simulink model "hydraulic_act_systems"  (R2013a)
settings: Solver=ode23t  StartTime=0.0  StopTime=10.0  FixedStep=1e-4  RelTol=1e-3
model workspace (MATLAB code in the model file):
  | % Data obtained from:
  | % ------------------------------------------------------------
  | % HyQ-Robot: Standard Definition for Joint Angles
  | % and Kinematic Parameters of the Legs and Torso
  | %
  | % Project: HyQ-Robot V1.0 with Leg V2.0
  | % Genoa, 9th July 2010
  | %-------------------------------------------------------------
  | % This Matlab file was made by:
  | % Job Ledezma
  | % Genova, Feb 2016
  | %-------------------------------------------------------------
  | 
  | 
  | % ________________________________________
  | %
  | %                HYL DESCRIPTION PARAMETERS
  | %________________________________________
  | 
  | % ---- Leg data ------
  | 
  | m1 = 1.772;              % Kg - Upper leg mass
  | m2 = 0.808;              % Kg - Lower leg mass
  | M = 3.982;                % Kg - Base mass
  | P_01 = 0.08;             % m - distance P0-P1
  | P_12 = 0.350;           % m - distance P1-P2
  | P_23 = 0.330;           % m - distance P2-P3
  | FR = 0.02;                 % m - foot radius
  | P1m1 = 0.164;           % m - distance P1-Pm1
  | P2m2 = 0.122;           % m - distance P2-Pm2
  | I1zz = 0.0713;           % kg·m2 - Inertia upper leg
  | I2zz = 0.0218;           % kg·m2 - Inertia lower leg
  | em1 = deg2rad(7.9);  % rad
  | em2 = deg2rad(0);     % rad
  | g  = 9.810;                 % m/s2 - gravity
  | 
  | % ----- Lever Arm Parameters -----
  | 
  | % Hip joint
  | a1   = 0.3219;             % m
  | b1   = 0.045;               % m
  | e11 = deg2rad(6.24); % rad
  | e12 = deg2rad(0);      % rad
  | 
  | % Knee joint
  | a2 = 0.3218;               % m
  | b2 = 0.045;                 % m
  | e21 = deg2rad(8.04);  % rad
  | e22 = deg2rad(6);       % rad
  | 
  | % ----- Limit Angles --------
  | 
  | % Initial conditions
  | q0_0 = 1;                           % m - height of the floating base
  | q1_0 = deg2rad(45);         % rad - HFE angle
  | q2_0 = deg2rad(-90);        % rad - KFE angle
  | 
  | % Max angle limits
  | q1Max = deg2rad(70);       % rad
  | q2Max = deg2rad(-20);      % rad
  | 
  | % Min angle limits
  | q1Min = deg2rad(-50);        % rad
  | q2Min = deg2rad(-140);      % rad
  | q0Min = P_01+P_12*cos(q1Min)+P_23*cos(q1Min+q2Min)+FR;     % m
  | 
  | % ________________________________________________________
  | %
  | %                                        HYDRAULIC PARAMETERS
  | % ________________________________________________________
  | 
  | % ------ Power unit --------
  | 
  | ps  = 160e5;                            % Pa - Supply pressure
  | pt  = 10e5;                              % Pa - Tank pressure
  | dpt = ps - pt;                           % Pa - Delta pressure
  | beta = 1.4e9;                          % Pa- Effective bulk modulus
  | 
  | % Initial condition for integrators
  | xo = 0;
  | 
  | pAo = 0;%ps/2;
  | pBo = 0;%ps/2;
  | 
  | %----- Cylinder - HOERBIGER LB6 16 10 0080 4M ----------
  | 
  | Dp = 0.016;                             % m - Piston diameter
  | Dr = 0.010;                              % m - Rod diameter
  | L  = 0.080;                               % m- Stroke
  | Aa = pi*(Dp^2)/4;                   % m^2 - Area A of the piston
  | Ab = pi*(Dp^2-Dr^2)/4;         % m^2 - Area B of the piston
  | r  = Aa/Ab;                              % Relation between areas
  | fv = 700;                                 %  Ns/m - Viscous friction
  | leak =1.7*10^-13;                 % m3/(s.Pa) - Cylinder leakage
  | Mp = ((pi*Dr^2/4)*L + Aa*0.15)*7860;    % Kg - Piston mass (approximated)
  | Lcyl = 0.280;                           % m - Total length of the cylinder
  | 
  | %-----  Valve Parameters - MOOG E024 - 177LA ----------
  | 
  | In   = 10;                               % I - Nominal control current
  | Qn   = 7.5 / 60e3;                 % m^3/s - Nominal flow rate
  | dptn = 70e5;                         % Pa - Valve pressure drop
  | Qlk   = 0.375 / 60e3;               % m^3/s - Leakage flow
  | Plk    = 70e5;                       % Pa - Nominal supply pressure for leakage test
  | wn    = 2*100*pi;                    % rad/s - Valve's natural frequency
  | E       = 0.7;                           % Valve's damping coefficient
  | Kv     = Qn/sqrt(dptn);          % m^3/(s*sqrt(Pa)) - Total flow coefficient
  | Kva    = Kv*sqrt(2);               % m^3/(s*sqrt(Pa)) - Partial flow coefficient A
  | Kvb    = Kv*sqrt(2);               % m^3/(s*sqrt(Pa)) - Partial flow coefficient B
  | Kvlk   = Qlk/sqrt(2*Plk);         % m^3/(s*sqrt(Pa)) - Total leakage flow coefficient
  | KvlkA  = Kvlk;                         % m^3/(s*sqrt(Pa)) -  Partial leakage flow coefficient A
  | KvlkB  = Kvlk;                         % m^3/(s*sqrt(Pa)) - Partial leakage flow coefficient B
  | up_dz = 0;                             % V - Upper limit of dead zone
  | lw_dz = 0;                              % V - Lower limit of dead zone
  | 
  | %------------   Manifold  -----------
  | % Review this part with the manifold's CAD design
  | 
  | v1a = (pi*(0.0035^2)/4)*0.07255;
  | v2a = (pi*(0.006^2)/4)*(0.090-0.012);
  | v1b = (pi*(0.0035^2)/4)*0.04491;
  | v2b = (pi*(0.006^2)/4)*(0.019+0.009);
  | v3b = (pi*(0.006^2)/4)*(0.007+0.009);
  | V0A = v1a + v2a;                                            % Dead volume coupled to chamber A
  | V0B = v1b + v2b + v3b;                                  % Dead volume coupled to chamber B
  | 
  | %-------  Load cell - BURSTER 8417-6005 ----------
  | 
  | xs = 20e-6;                            % m - Maximum deflection @ full scale
  | Fs = 5000;                             % N - Maximum force
  | Ks = Fs / xs ;                         % N·m - Load cell stiffness
  | 
  | noise = 0;                            %N - noise due nonlinearities, hysteresis, non repeatibility
  | 
  | %------ Accumulator - FOX-ITALY HST 0,04 ----------
  | 
  | acc = 0;
  | 
  | n = 1.4;                                % Polytropic constant
  | V0 = 0.04e-3;                       % m3 - Initial volume
  | P0 = 100e5 + 1e5;               % Pa - Precharge pressure
libraries: sdolib x4
settings Model: Creator=Toshiba  LastModifiedBy=Toshiba
settings SolverCC: ZeroCrossAlgorithm=Adaptive

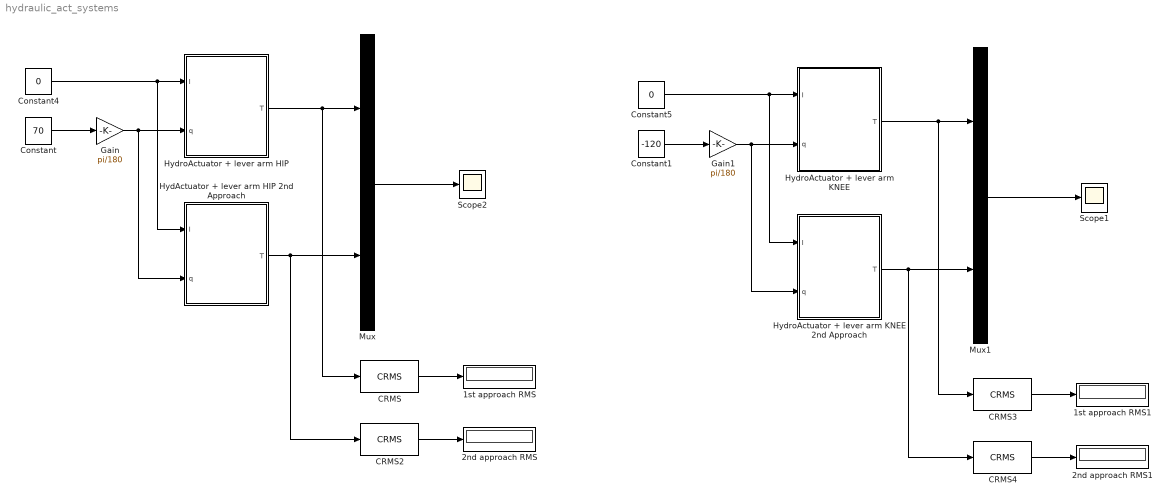
== system hydraulic_act_systems ==
  1st approach RMS : Display
  1st approach RMS1 : Display
  2nd approach RMS : Display
  2nd approach RMS1 : Display
  CRMS{,2..4} (4 alike) : sdolib/RMS Blocks/CRMS
  Constant : Constant  Value=70
  Constant1 : Constant  Value=-120
  Constant4 : Constant  Value=0
  Constant5 : Constant  Value=0
  Gain : Gain  Gain=pi/180
  Gain1 : Gain  Gain=pi/180
  HydActuator + lever arm HIP 2nd Approach : Subsystem
  HydroActuator + lever arm HIP : Subsystem
  HydroActuator + lever arm KNEE : Subsystem
  HydroActuator + lever arm KNEE 2nd Approach : Subsystem
  Mux : Mux  Inputs=2
  Mux1 : Mux  Inputs=2
  Scope1 : Scope
      settings: YMin=-152500  YMax=-117500
  Scope2 : Scope
      settings: YMin=-152500  YMax=-117500  SaveName=ScopeData2
  wires:
  Constant/1 -> Gain/1
  Gain/1 -> HydActuator + lever arm HIP 2nd Approach/2(q), HydroActuator + lever arm HIP/2(q)
  Constant1/1 -> Gain1/1
  Gain1/1 -> HydroActuator + lever arm KNEE 2nd Approach/2(q), HydroActuator + lever arm KNEE/2(q)
  Constant4/1 -> HydActuator + lever arm HIP 2nd Approach/1(I), HydroActuator + lever arm HIP/1(I)
  Constant5/1 -> HydroActuator + lever arm KNEE 2nd Approach/1(I), HydroActuator + lever arm KNEE/1(I)
  HydroActuator + lever arm HIP/1(T) -> CRMS/1, Mux/1
  HydActuator + lever arm HIP 2nd Approach/1(T) -> CRMS2/1, Mux/2
  Mux/1 -> Scope2/1
  HydroActuator + lever arm KNEE/1(T) -> CRMS3/1, Mux1/1
  HydroActuator + lever arm KNEE 2nd Approach/1(T) -> CRMS4/1, Mux1/2
  CRMS/1 -> 1st approach RMS/1
  Mux1/1 -> Scope1/1
  CRMS2/1 -> 2nd approach RMS/1
  CRMS3/1 -> 1st approach RMS1/1
  CRMS4/1 -> 2nd approach RMS1/1

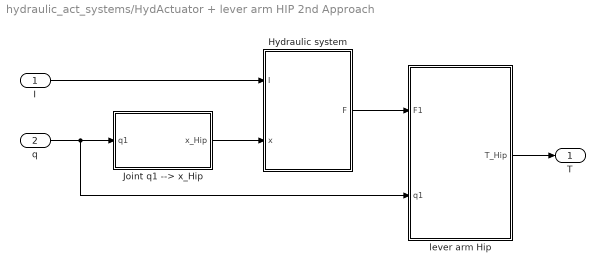
== system hydraulic_act_systems/HydActuator + lever arm HIP 2nd Approach ==
  I : Inport
  q : Inport  Port=2
  Hydraulic system : Subsystem
  "Joint q1 --> x_Hip  " : MATLAB Function  TreatAsAtomicUnit=on
  lever arm Hip : MATLAB Function  TreatAsAtomicUnit=on
  T : Outport
  wires:
  q/1 -> "Joint q1 --> x_Hip  "/1(q1), lever arm Hip/2(q1)
  I/1 -> Hydraulic system/1(I)
  lever arm Hip/1(T_Hip) -> T/1
  Hydraulic system/1(F) -> lever arm Hip/1(F1)
  "Joint q1 --> x_Hip  "/1(x_Hip) -> Hydraulic system/2(x)

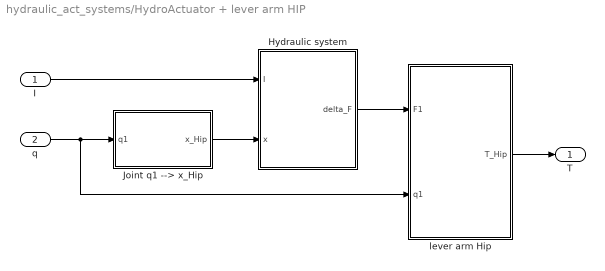
== system hydraulic_act_systems/HydroActuator + lever arm HIP ==
  I : Inport
  q : Inport  Port=2
  Hydraulic system : Subsystem
  "Joint q1 --> x_Hip  " : MATLAB Function  TreatAsAtomicUnit=on
  lever arm Hip : MATLAB Function  TreatAsAtomicUnit=on
  T : Outport
  wires:
  "Joint q1 --> x_Hip  "/1(x_Hip) -> Hydraulic system/2(x)
  Hydraulic system/1(delta_F) -> lever arm Hip/1(F1)
  lever arm Hip/1(T_Hip) -> T/1
  I/1 -> Hydraulic system/1(I)
  q/1 -> lever arm Hip/2(q1), "Joint q1 --> x_Hip  "/1(q1)

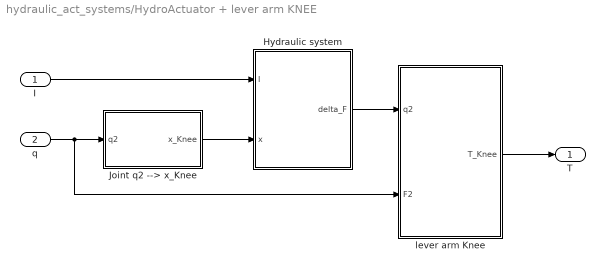
== system hydraulic_act_systems/HydroActuator + lever arm KNEE ==
  I : Inport
  q : Inport  Port=2
  Hydraulic system : Subsystem
  Joint q2 --> x_Knee : MATLAB Function  TreatAsAtomicUnit=on
  lever arm Knee : MATLAB Function  TreatAsAtomicUnit=on
  T : Outport
  wires:
  q/1 -> lever arm Knee/2(F2), Joint q2 --> x_Knee/1(q2)
  Joint q2 --> x_Knee/1(x_Knee) -> Hydraulic system/2(x)
  Hydraulic system/1(delta_F) -> lever arm Knee/1(q2)
  I/1 -> Hydraulic system/1(I)
  lever arm Knee/1(T_Knee) -> T/1

== system hydraulic_act_systems/HydroActuator + lever arm KNEE 2nd Approach ==
  I : Inport
  q : Inport  Port=2
  Hydraulic system : Subsystem
  Joint q2 --> x_Knee : MATLAB Function  TreatAsAtomicUnit=on
  lever arm Knee : MATLAB Function  TreatAsAtomicUnit=on
  T : Outport
  wires:
  lever arm Knee/1(T_Knee) -> T/1
  I/1 -> Hydraulic system/1(I)
  Hydraulic system/1(F) -> lever arm Knee/1(q2)
  Joint q2 --> x_Knee/1(x_Knee) -> Hydraulic system/2(x)
  q/1 -> Joint q2 --> x_Knee/1(q2), lever arm Knee/2(F2)

== system hydraulic_act_systems/HydActuator + lever arm HIP 2nd Approach/Hydraulic system ==
  I : Inport
  x : Inport  Port=2
  Cylinder HOERBIGER LB6 1610 0080 4M : Subsystem
  Servovalve MOOG E024-177LA : Subsystem
  F : Outport
  wires:
  Servovalve MOOG E024-177LA/2(qB) -> Cylinder HOERBIGER LB6 1610 0080 4M/2(qB)
  Servovalve MOOG E024-177LA/1(qA) -> Cylinder HOERBIGER LB6 1610 0080 4M/1(qA)
  Cylinder HOERBIGER LB6 1610 0080 4M/2(pA) -> Servovalve MOOG E024-177LA/2(pA)
  Cylinder HOERBIGER LB6 1610 0080 4M/3(pB) -> Servovalve MOOG E024-177LA/3(pB)
  I/1 -> Servovalve MOOG E024-177LA/1(I)
  Cylinder HOERBIGER LB6 1610 0080 4M/1(F) -> F/1
  x/1 -> Cylinder HOERBIGER LB6 1610 0080 4M/3(x)

== system hydraulic_act_systems/HydroActuator + lever arm HIP/Hydraulic system ==
  I : Inport
  x : Inport  Port=2
  Cylinder HOERBIGER LB6 1610 0080 4M : Subsystem
  Servovalve MOOG E024-177LA : Subsystem
  delta_F : Outport
  wires:
  Servovalve MOOG E024-177LA/2(qB) -> Cylinder HOERBIGER LB6 1610 0080 4M/2(qB)
  Servovalve MOOG E024-177LA/1(qA) -> Cylinder HOERBIGER LB6 1610 0080 4M/1(qA)
  Cylinder HOERBIGER LB6 1610 0080 4M/2(pA1) -> Servovalve MOOG E024-177LA/2(pA)
  Cylinder HOERBIGER LB6 1610 0080 4M/3(pB1) -> Servovalve MOOG E024-177LA/3(pB)
  I/1 -> Servovalve MOOG E024-177LA/1(I)
  Cylinder HOERBIGER LB6 1610 0080 4M/1(delta_F) -> delta_F/1
  x/1 -> Cylinder HOERBIGER LB6 1610 0080 4M/3(x)

== system hydraulic_act_systems/HydroActuator + lever arm KNEE/Hydraulic system ==
  I : Inport
  x : Inport  Port=2
  Cylinder HOERBIGER LB6 1610 0080 4M : Subsystem
  Servovalve MOOG E024-177LA : Subsystem
  delta_F : Outport
  wires:
  Servovalve MOOG E024-177LA/2(qB) -> Cylinder HOERBIGER LB6 1610 0080 4M/2(qB)
  Servovalve MOOG E024-177LA/1(qA) -> Cylinder HOERBIGER LB6 1610 0080 4M/1(qA)
  Cylinder HOERBIGER LB6 1610 0080 4M/2(pA1) -> Servovalve MOOG E024-177LA/2(pA)
  Cylinder HOERBIGER LB6 1610 0080 4M/3(pB1) -> Servovalve MOOG E024-177LA/3(pB)
  I/1 -> Servovalve MOOG E024-177LA/1(I)
  Cylinder HOERBIGER LB6 1610 0080 4M/1(delta_F) -> delta_F/1
  x/1 -> Cylinder HOERBIGER LB6 1610 0080 4M/3(x)

== system hydraulic_act_systems/HydroActuator + lever arm KNEE 2nd Approach/Hydraulic system ==
  I : Inport
  x : Inport  Port=2
  Cylinder HOERBIGER LB6 1610 0080 4M : Subsystem
  Servovalve MOOG E024-177LA : Subsystem
  F : Outport
  wires:
  Servovalve MOOG E024-177LA/2(qB) -> Cylinder HOERBIGER LB6 1610 0080 4M/2(qB)
  Servovalve MOOG E024-177LA/1(qA) -> Cylinder HOERBIGER LB6 1610 0080 4M/1(qA)
  Cylinder HOERBIGER LB6 1610 0080 4M/2(pA) -> Servovalve MOOG E024-177LA/2(pA)
  Cylinder HOERBIGER LB6 1610 0080 4M/3(pB) -> Servovalve MOOG E024-177LA/3(pB)
  I/1 -> Servovalve MOOG E024-177LA/1(I)
  Cylinder HOERBIGER LB6 1610 0080 4M/1(F) -> F/1
  x/1 -> Cylinder HOERBIGER LB6 1610 0080 4M/3(x)

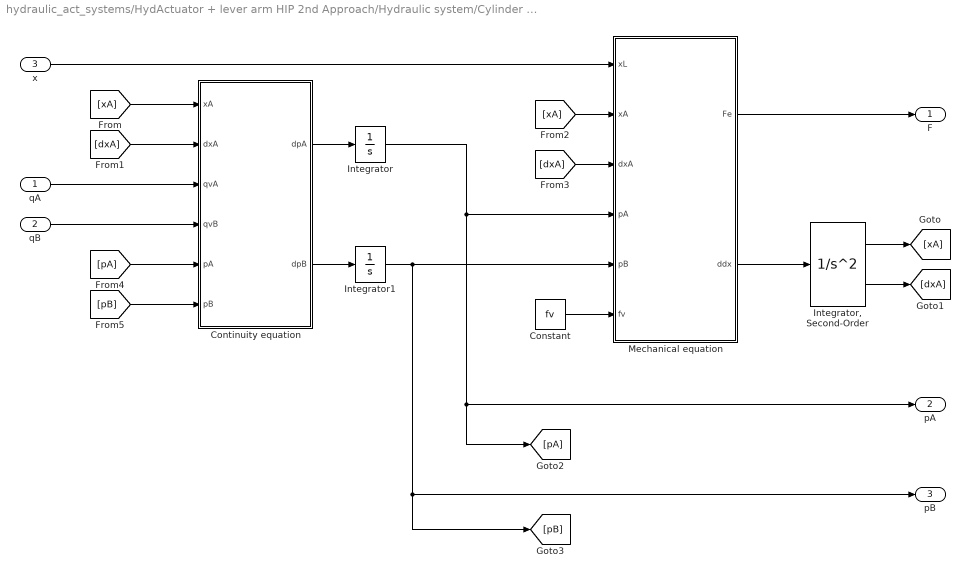
== system hydraulic_act_systems/HydActuator + lever arm HIP 2nd Approach/Hydraulic system/Cylinder HOERBIGER LB6 1610 0080 4M ==
  qA : Inport
  qB : Inport  Port=2
  x : Inport  Port=3
  Constant : Constant  Value=fv
  Continuity equation : MATLAB Function  TreatAsAtomicUnit=on
  Integrator : Integrator  InitialCondition=pAo
  "Integrator, Second-Order" : SecondOrderIntegrator  ICX=xo  LimitX=on  UpperLimitX=L  LowerLimitX=0
  Integrator1 : Integrator  InitialCondition=pBo
  Mechanical equation : MATLAB Function  TreatAsAtomicUnit=on
  F : Outport
  pA : Outport  Port=2
  pB : Outport  Port=3
  wires:
  Continuity equation/1(dpA) -> Integrator/1
  Continuity equation/2(dpB) -> Integrator1/1
  Integrator/1 -> [pA], pA/1, Mechanical equation/4(pA)
  Integrator1/1 -> pB/1, [pB], Mechanical equation/5(pB)
  qA/1 -> Continuity equation/3(qvA)
  qB/1 -> Continuity equation/4(qvB)
  Mechanical equation/2(ddx) -> "Integrator, Second-Order"/1
  [dxA] -> Continuity equation/2(dxA)
  [xA] -> Continuity equation/1(xA)
  "Integrator, Second-Order"/1 -> [xA]
  "Integrator, Second-Order"/2 -> [dxA]
  Constant/1 -> Mechanical equation/6(fv)
  [xA] -> Mechanical equation/2(xA)
  [dxA] -> Mechanical equation/3(dxA)
  [pA] -> Continuity equation/5(pA)
  [pB] -> Continuity equation/6(pB)
  Mechanical equation/1(Fe) -> F/1
  x/1 -> Mechanical equation/1(xL)

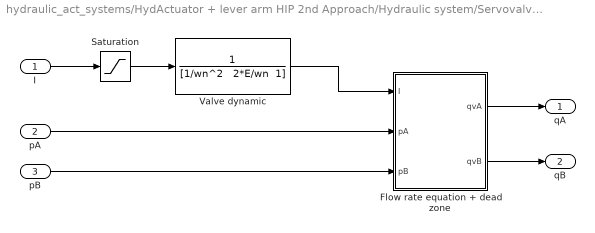
== system hydraulic_act_systems/HydActuator + lever arm HIP 2nd Approach/Hydraulic system/Servovalve MOOG E024-177LA ==
  I : Inport
  pA : Inport  Port=2
  pB : Inport  Port=3
  Flow rate equation + dead zone : MATLAB Function  TreatAsAtomicUnit=on
  Saturation : Saturate  UpperLimit=In  LowerLimit=-In  LinearizeAsGain=off
  Valve dynamic : TransferFcn  Numerator=1  Denominator="[1/wn^2   2*E/wn  1]"
  qA : Outport
  qB : Outport  Port=2
  wires:
  Saturation/1 -> Valve dynamic/1
  I/1 -> Saturation/1
  Valve dynamic/1 -> Flow rate equation + dead zone/1(I)
  pA/1 -> Flow rate equation + dead zone/2(pA)
  pB/1 -> Flow rate equation + dead zone/3(pB)
  Flow rate equation + dead zone/2(qvB) -> qB/1
  Flow rate equation + dead zone/1(qvA) -> qA/1

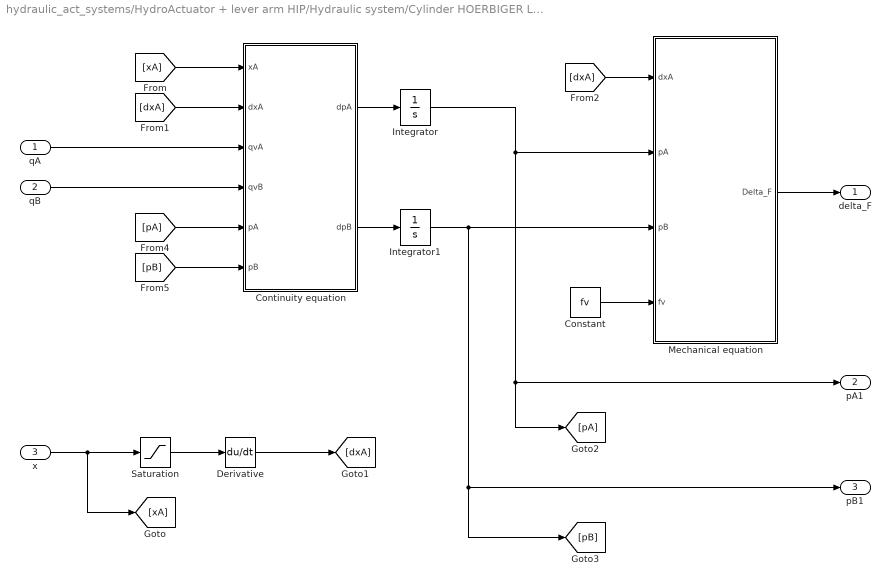
== system hydraulic_act_systems/HydroActuator + lever arm HIP/Hydraulic system/Cylinder HOERBIGER LB6 1610 0080 4M ==
  qA : Inport
  qB : Inport  Port=2
  x : Inport  Port=3
  Constant : Constant  Value=fv
  Continuity equation : MATLAB Function  TreatAsAtomicUnit=on
  Derivative : Derivative
  Integrator : Integrator  InitialCondition=pAo
  Integrator1 : Integrator  InitialCondition=pBo
  Mechanical equation : MATLAB Function  TreatAsAtomicUnit=on
  Saturation : Saturate  UpperLimit=L  LowerLimit=0
  delta_F : Outport
  pA1 : Outport  Port=2
  pB1 : Outport  Port=3
  wires:
  Continuity equation/1(dpA) -> Integrator/1
  Continuity equation/2(dpB) -> Integrator1/1
  qA/1 -> Continuity equation/3(qvA)
  qB/1 -> Continuity equation/4(qvB)
  [dxA] -> Continuity equation/2(dxA)
  [xA] -> Continuity equation/1(xA)
  Constant/1 -> Mechanical equation/4(fv)
  Derivative/1 -> [dxA]
  Mechanical equation/1(Delta_F) -> delta_F/1
  x/1 -> [xA], Saturation/1
  Saturation/1 -> Derivative/1
  [dxA] -> Mechanical equation/1(dxA)
  Integrator/1 -> [pA], pA1/1, Mechanical equation/2(pA)
  Integrator1/1 -> [pB], pB1/1, Mechanical equation/3(pB)
  [pA] -> Continuity equation/5(pA)
  [pB] -> Continuity equation/6(pB)

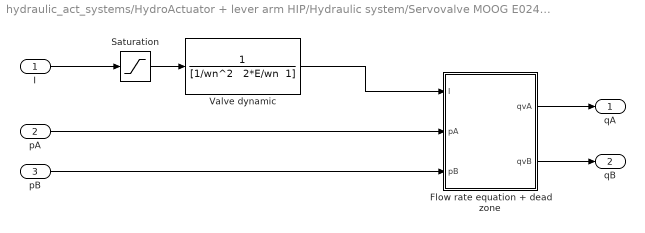
== system hydraulic_act_systems/HydroActuator + lever arm HIP/Hydraulic system/Servovalve MOOG E024-177LA ==
  I : Inport
  pA : Inport  Port=2
  pB : Inport  Port=3
  Flow rate equation + dead zone : MATLAB Function  TreatAsAtomicUnit=on
  Saturation : Saturate  UpperLimit=In  LowerLimit=-In  LinearizeAsGain=off
  Valve dynamic : TransferFcn  Numerator=1  Denominator="[1/wn^2   2*E/wn  1]"
  qA : Outport
  qB : Outport  Port=2
  wires:
  Saturation/1 -> Valve dynamic/1
  I/1 -> Saturation/1
  Valve dynamic/1 -> Flow rate equation + dead zone/1(I)
  pA/1 -> Flow rate equation + dead zone/2(pA)
  pB/1 -> Flow rate equation + dead zone/3(pB)
  Flow rate equation + dead zone/2(qvB) -> qB/1
  Flow rate equation + dead zone/1(qvA) -> qA/1

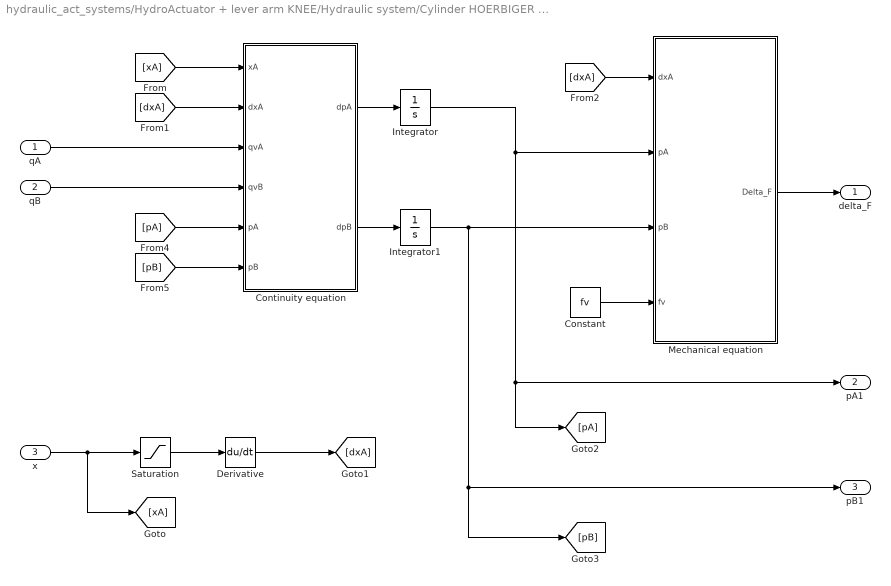
== system hydraulic_act_systems/HydroActuator + lever arm KNEE/Hydraulic system/Cylinder HOERBIGER LB6 1610 0080 4M ==
  qA : Inport
  qB : Inport  Port=2
  x : Inport  Port=3
  Constant : Constant  Value=fv
  Continuity equation : MATLAB Function  TreatAsAtomicUnit=on
  Derivative : Derivative
  Integrator : Integrator  InitialCondition=pAo
  Integrator1 : Integrator  InitialCondition=pBo
  Mechanical equation : MATLAB Function  TreatAsAtomicUnit=on
  Saturation : Saturate  UpperLimit=L  LowerLimit=0
  delta_F : Outport
  pA1 : Outport  Port=2
  pB1 : Outport  Port=3
  wires:
  Continuity equation/1(dpA) -> Integrator/1
  Continuity equation/2(dpB) -> Integrator1/1
  qA/1 -> Continuity equation/3(qvA)
  qB/1 -> Continuity equation/4(qvB)
  [dxA] -> Continuity equation/2(dxA)
  [xA] -> Continuity equation/1(xA)
  Constant/1 -> Mechanical equation/4(fv)
  Derivative/1 -> [dxA]
  Mechanical equation/1(Delta_F) -> delta_F/1
  x/1 -> [xA], Saturation/1
  Saturation/1 -> Derivative/1
  [dxA] -> Mechanical equation/1(dxA)
  Integrator/1 -> [pA], pA1/1, Mechanical equation/2(pA)
  Integrator1/1 -> [pB], pB1/1, Mechanical equation/3(pB)
  [pA] -> Continuity equation/5(pA)
  [pB] -> Continuity equation/6(pB)

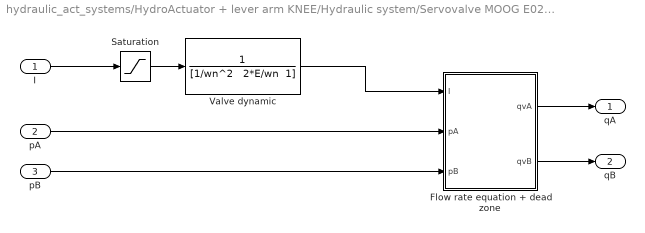
== system hydraulic_act_systems/HydroActuator + lever arm KNEE/Hydraulic system/Servovalve MOOG E024-177LA ==
  I : Inport
  pA : Inport  Port=2
  pB : Inport  Port=3
  Flow rate equation + dead zone : MATLAB Function  TreatAsAtomicUnit=on
  Saturation : Saturate  UpperLimit=In  LowerLimit=-In  LinearizeAsGain=off
  Valve dynamic : TransferFcn  Numerator=1  Denominator="[1/wn^2   2*E/wn  1]"
  qA : Outport
  qB : Outport  Port=2
  wires:
  Saturation/1 -> Valve dynamic/1
  I/1 -> Saturation/1
  Valve dynamic/1 -> Flow rate equation + dead zone/1(I)
  pA/1 -> Flow rate equation + dead zone/2(pA)
  pB/1 -> Flow rate equation + dead zone/3(pB)
  Flow rate equation + dead zone/2(qvB) -> qB/1
  Flow rate equation + dead zone/1(qvA) -> qA/1

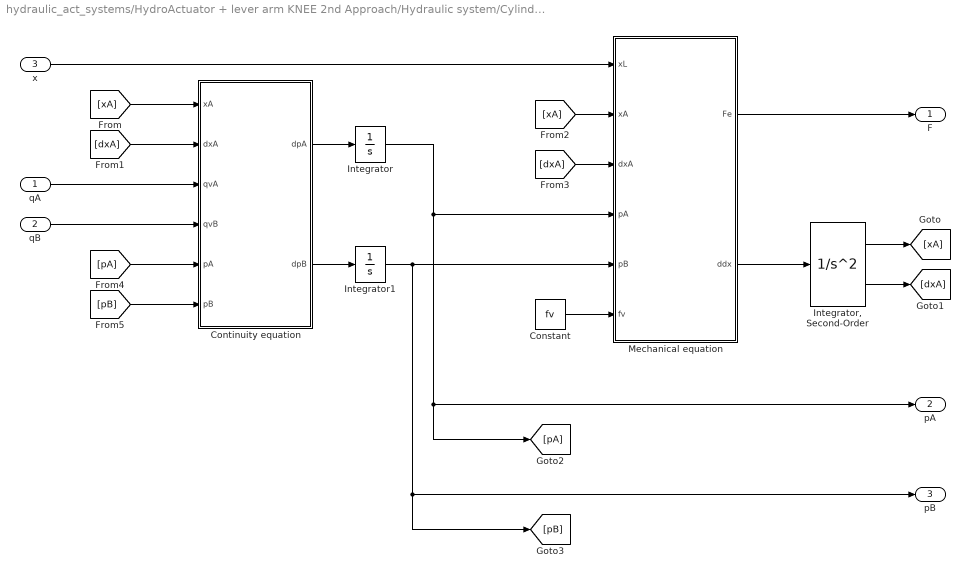
== system hydraulic_act_systems/HydroActuator + lever arm KNEE 2nd Approach/Hydraulic system/Cylinder HOERBIGER LB6 1610 0080 4M ==
  qA : Inport
  qB : Inport  Port=2
  x : Inport  Port=3
  Constant : Constant  Value=fv
  Continuity equation : MATLAB Function  TreatAsAtomicUnit=on
  Integrator : Integrator  InitialCondition=pAo
  "Integrator, Second-Order" : SecondOrderIntegrator  ICX=xo  LimitX=on  UpperLimitX=L  LowerLimitX=0
  Integrator1 : Integrator  InitialCondition=pBo
  Mechanical equation : MATLAB Function  TreatAsAtomicUnit=on
  F : Outport
  pA : Outport  Port=2
  pB : Outport  Port=3
  wires:
  Continuity equation/1(dpA) -> Integrator/1
  Continuity equation/2(dpB) -> Integrator1/1
  Integrator/1 -> [pA], pA/1, Mechanical equation/4(pA)
  Integrator1/1 -> pB/1, [pB], Mechanical equation/5(pB)
  qA/1 -> Continuity equation/3(qvA)
  qB/1 -> Continuity equation/4(qvB)
  Mechanical equation/2(ddx) -> "Integrator, Second-Order"/1
  [dxA] -> Continuity equation/2(dxA)
  [xA] -> Continuity equation/1(xA)
  "Integrator, Second-Order"/1 -> [xA]
  "Integrator, Second-Order"/2 -> [dxA]
  Constant/1 -> Mechanical equation/6(fv)
  [xA] -> Mechanical equation/2(xA)
  [dxA] -> Mechanical equation/3(dxA)
  [pA] -> Continuity equation/5(pA)
  [pB] -> Continuity equation/6(pB)
  Mechanical equation/1(Fe) -> F/1
  x/1 -> Mechanical equation/1(xL)

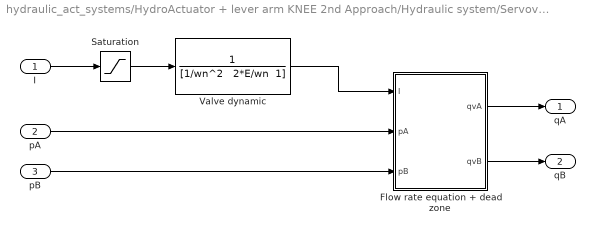
== system hydraulic_act_systems/HydroActuator + lever arm KNEE 2nd Approach/Hydraulic system/Servovalve MOOG E024-177LA ==
  I : Inport
  pA : Inport  Port=2
  pB : Inport  Port=3
  Flow rate equation + dead zone : MATLAB Function  TreatAsAtomicUnit=on
  Saturation : Saturate  UpperLimit=In  LowerLimit=-In  LinearizeAsGain=off
  Valve dynamic : TransferFcn  Numerator=1  Denominator="[1/wn^2   2*E/wn  1]"
  qA : Outport
  qB : Outport  Port=2
  wires:
  Saturation/1 -> Valve dynamic/1
  I/1 -> Saturation/1
  Valve dynamic/1 -> Flow rate equation + dead zone/1(I)
  pA/1 -> Flow rate equation + dead zone/2(pA)
  pB/1 -> Flow rate equation + dead zone/3(pB)
  Flow rate equation + dead zone/2(qvB) -> qB/1
  Flow rate equation + dead zone/1(qvA) -> qA/1

== matlab function hydraulic_act_systems/HydActuator + lever arm HIP 2nd Approach/Hydraulic system/Cylinder HOERBIGER LB6 1610 0080 4M/Continuity equation ==
  data: xA input; dpA output; dpB output; dxA input; qvA input; qvB input; pA input; pB input; leak parameter; V0A parameter; V0B parameter; Aa parameter; Ab parameter; L parameter; beta parameter; n parameter; V0 parameter; P0 parameter; acc parameter
function [dpA,dpB] = fcn(xA, dxA, qvA, qvB, pA, pB, leak, V0A, V0B, Aa, Ab, L, beta, n, V0, P0, acc)

pC = pA - pB;   % Pressao de carga [Pa]

qvlk = leak * pC;
dpa = 0;
dpb = 0;

if acc == 0,
%       /              \
%       |     beta     | /                    \
% dpA = | ------------ | | qvA - Aa*dx - qvex | 
%       |  Va0 + Aa*x  | \                    /
%       \              /
      
dpa = (beta/(V0A + Aa*xA)) * (qvA - Aa*dxA - qvlk);

%       /                  \
%       |     beta         | /                    \
% dpB = | ---------------- | | Ab*dx + qvex - qvB | 
%       | Vb0 + Ab*(L - x) | \                    /
%       \                  /
      
dpb = (beta/(V0B + Ab*(L-xA))) * (Ab*dxA + qvlk - qvB);

elseif acc == 1,
    
CA_A  = (V0A + Aa*xA) / beta;                      % Capacitancia hidráulica do atuador [m^3/Pa]
CAC_A = (V0*P0^(1/n))/(n* (pA+1e5)^((n+1)/n));     % Capacitancia hidráulica do acumulador [m^3/Pa]
CA_B  = (V0B + Ab*(L-xA)) / beta;                  % Capacitancia hidráulica do atuador [m^3/Pa]
CAC_B = (V0*P0^(1/n))/(n* (pB+1e5)^((n+1)/n));     % Capacitancia hidráulica do acumulador [m^3/Pa]

CT_A  = CA_A + CAC_A;                              % Capacitancia total em A
CT_B  = CA_B + CAC_B;                              % Capacitancia total em B 


%       /        \
%       |   1    | /                    \
% dpA = | ------ | | qvA - Aa*dx - qvex | 
%       |  CT_A  | \                    /
%       \        /
      
dpa = CT_A^-1 * (qvA - Aa*dxA - qvlk);

%       /        \
%       |   1    | /                    \
% dpB = | ------ | | Ab*dx + qvex - qvB | 
%       |  CT_B  | \                    /
%       \        /
      
dpb = CT_B^-1 * (Ab*dxA + qvlk - qvB);
end

dpA = dpa;
dpB = dpb;

== matlab function hydraulic_act_systems/HydActuator + lever arm HIP 2nd Approach/Hydraulic system/Cylinder HOERBIGER LB6 1610 0080 4M/Mechanical equation ==
  data: Fe output; xL input; xA input; dxA input; ddx output; pA input; pB input; fv input; Aa parameter; Ab parameter; Ks parameter; Mp parameter; noise parameter
function [Fe, ddx] = fcn(xL, xA, dxA, pA, pB, fv, Aa, Ab, Ks, Mp, noise)
%#codegen

FH  = pA*Aa - pB*Ab;                % N - Hydraulic force
Ffr = fv*dxA;                       % N - Friction force (Viscous)
Fe  = Ks*(xA - xL) + noise*randn(1);% N - Force measured by the sensor + noise
ddx = (FH - Ffr - Fe)/Mp;        % m/s2 - Acceleration

== matlab function hydraulic_act_systems/HydroActuator + lever arm HIP/Hydraulic system/Cylinder HOERBIGER LB6 1610 0080 4M/Continuity equation ==
  data: xA input; dpA output; dpB output; dxA input; qvA input; qvB input; pA input; pB input; leak parameter; V0A parameter; V0B parameter; Aa parameter; Ab parameter; L parameter; beta parameter; n parameter; V0 parameter; P0 parameter; acc parameter
function [dpA,dpB] = fcn(xA, dxA, qvA, qvB, pA, pB, leak, V0A, V0B, Aa, Ab, L, beta, n, V0, P0, acc)

pC = pA - pB;   % Pressao de carga [Pa]

qvlk = leak * pC;
dpa = 0;
dpb = 0;

if acc == 0,
%       /              \
%       |     beta     | /                    \
% dpA = | ------------ | | qvA - Aa*dx - qvex | 
%       |  Va0 + Aa*x  | \                    /
%       \              /
      
dpa = (beta/(V0A + Aa*xA)) * (qvA - Aa*dxA - qvlk);

%       /                  \
%       |     beta         | /                    \
% dpB = | ---------------- | | Ab*dx + qvex - qvB | 
%       | Vb0 + Ab*(L - x) | \                    /
%       \                  /
      
dpb = (beta/(V0B + Ab*(L-xA))) * (Ab*dxA + qvlk - qvB);

elseif acc == 1,
    
CA_A  = (V0A + Aa*xA) / beta;                      % Capacitancia hidráulica do atuador [m^3/Pa]
CAC_A = (V0*P0^(1/n))/(n* (pA+1e5)^((n+1)/n));     % Capacitancia hidráulica do acumulador [m^3/Pa]
CA_B  = (V0B + Ab*(L-xA)) / beta;                  % Capacitancia hidráulica do atuador [m^3/Pa]
CAC_B = (V0*P0^(1/n))/(n* (pB+1e5)^((n+1)/n));     % Capacitancia hidráulica do acumulador [m^3/Pa]

CT_A  = CA_A + CAC_A;                              % Capacitancia total em A
CT_B  = CA_B + CAC_B;                              % Capacitancia total em B 


%       /        \
%       |   1    | /                    \
% dpA = | ------ | | qvA - Aa*dx - qvex | 
%       |  CT_A  | \                    /
%       \        /
      
dpa = CT_A^-1 * (qvA - Aa*dxA - qvlk);

%       /        \
%       |   1    | /                    \
% dpB = | ------ | | Ab*dx + qvex - qvB | 
%       |  CT_B  | \                    /
%       \        /
      
dpb = CT_B^-1 * (Ab*dxA + qvlk - qvB);
end

dpA = dpa;
dpB = dpb;

== matlab function hydraulic_act_systems/HydroActuator + lever arm HIP/Hydraulic system/Cylinder HOERBIGER LB6 1610 0080 4M/Mechanical equation ==
  data: Delta_F output; dxA input; pA input; pB input; fv input; Aa parameter; Ab parameter
function Delta_F = fcn(dxA, pA, pB, fv, Aa, Ab)
%#codegen

FH  = pA*Aa - pB*Ab;     % N - Hydraulic force
Ffr = fv*dxA;            % N - Friction force (Viscous)
Delta_F  = FH - Ffr;     % m/s2 - Acceleration

== matlab function hydraulic_act_systems/HydActuator + lever arm HIP 2nd Approach/Hydraulic system/Servovalve MOOG E024-177LA/Flow rate equation + dead zone ==
  data I settings: updateMethod=SF_CONTINUOUS_TIME_DATA
  data qvA settings: updateMethod=SF_CONTINUOUS_TIME_DATA
  data qvB settings: updateMethod=SF_CONTINUOUS_TIME_DATA
  data: I input; qvA output; qvB output; In parameter; Kva parameter; Kvb parameter; KvlkA parameter; KvlkB parameter; up_dz parameter; lw_dz parameter; ps parameter; pt parameter; pA input; pB input
function [qvA , qvB] = fcn(I, In, Kva, Kvb, KvlkA, KvlkB,up_dz, lw_dz, ps, pt, pA, pB)

if (I>=up_dz) && (I<=In),
    qvA = (Kva*(I/In) + KvlkA) * sign(ps-pA)*sqrt(abs(ps-pA)) - KvlkA*sign(pA-pt)*sqrt(abs(pA-pt)) ;
    qvB = (Kvb*(I/In) + KvlkB) * sign(pB-pt)*sqrt(abs(pB-pt)) - KvlkB*sign(ps-pB)*sqrt(abs(ps-pB)) ;
elseif (I>=-In) && (I<=lw_dz), 
    qvA = KvlkA*sign(ps-pA)*sqrt(abs(ps-pA)) - (Kva*(abs(I)/In) + KvlkA) * sign(pA-pt)*sqrt(abs(pA-pt));
     qvB = KvlkB*sign(pB-pt)*sqrt(abs(pB-pt)) - (Kvb*(abs(I)/In) + KvlkB) * sign(ps-pB)*sqrt(abs(ps-pB));
else
    qvA = 0;
    qvB = 0;
end
end

== matlab function hydraulic_act_systems/HydroActuator + lever arm HIP/Hydraulic system/Servovalve MOOG E024-177LA/Flow rate equation + dead zone ==
  data I settings: updateMethod=SF_CONTINUOUS_TIME_DATA
  data qvA settings: updateMethod=SF_CONTINUOUS_TIME_DATA
  data qvB settings: updateMethod=SF_CONTINUOUS_TIME_DATA
  data: I input; qvA output; qvB output; In parameter; Kva parameter; Kvb parameter; KvlkA parameter; KvlkB parameter; up_dz parameter; lw_dz parameter; ps parameter; pt parameter; pA input; pB input
function [qvA , qvB] = fcn(I, In, Kva, Kvb, KvlkA, KvlkB,up_dz, lw_dz, ps, pt, pA, pB)

if (I>=up_dz) && (I<=In),
    qvA = (Kva*(I/In) + KvlkA) * sign(ps-pA)*sqrt(abs(ps-pA)) - KvlkA*sign(pA-pt)*sqrt(abs(pA-pt)) ;
    qvB = (Kvb*(I/In) + KvlkB) * sign(pB-pt)*sqrt(abs(pB-pt)) - KvlkB*sign(ps-pB)*sqrt(abs(ps-pB)) ;
elseif (I>=-In) && (I<=lw_dz), 
    qvA = KvlkA*sign(ps-pA)*sqrt(abs(ps-pA)) - (Kva*(abs(I)/In) + KvlkA) * sign(pA-pt)*sqrt(abs(pA-pt));
     qvB = KvlkB*sign(pB-pt)*sqrt(abs(pB-pt)) - (Kvb*(abs(I)/In) + KvlkB) * sign(ps-pB)*sqrt(abs(ps-pB));
else
    qvA = 0;
    qvB = 0;
end
end

== matlab function hydraulic_act_systems/HydroActuator + lever arm KNEE/Hydraulic system/Cylinder HOERBIGER LB6 1610 0080 4M/Continuity equation ==
  data: xA input; dpA output; dpB output; dxA input; qvA input; qvB input; pA input; pB input; leak parameter; V0A parameter; V0B parameter; Aa parameter; Ab parameter; L parameter; beta parameter; n parameter; V0 parameter; P0 parameter; acc parameter
function [dpA,dpB] = fcn(xA, dxA, qvA, qvB, pA, pB, leak, V0A, V0B, Aa, Ab, L, beta, n, V0, P0, acc)

pC = pA - pB;   % Pressao de carga [Pa]

qvlk = leak * pC;
dpa = 0;
dpb = 0;

if acc == 0,
%       /              \
%       |     beta     | /                    \
% dpA = | ------------ | | qvA - Aa*dx - qvex | 
%       |  Va0 + Aa*x  | \                    /
%       \              /
      
dpa = (beta/(V0A + Aa*xA)) * (qvA - Aa*dxA - qvlk);

%       /                  \
%       |     beta         | /                    \
% dpB = | ---------------- | | Ab*dx + qvex - qvB | 
%       | Vb0 + Ab*(L - x) | \                    /
%       \                  /
      
dpb = (beta/(V0B + Ab*(L-xA))) * (Ab*dxA + qvlk - qvB);

elseif acc == 1,
    
CA_A  = (V0A + Aa*xA) / beta;                      % Capacitancia hidráulica do atuador [m^3/Pa]
CAC_A = (V0*P0^(1/n))/(n* (pA+1e5)^((n+1)/n));     % Capacitancia hidráulica do acumulador [m^3/Pa]
CA_B  = (V0B + Ab*(L-xA)) / beta;                  % Capacitancia hidráulica do atuador [m^3/Pa]
CAC_B = (V0*P0^(1/n))/(n* (pB+1e5)^((n+1)/n));     % Capacitancia hidráulica do acumulador [m^3/Pa]

CT_A  = CA_A + CAC_A;                              % Capacitancia total em A
CT_B  = CA_B + CAC_B;                              % Capacitancia total em B 


%       /        \
%       |   1    | /                    \
% dpA = | ------ | | qvA - Aa*dx - qvex | 
%       |  CT_A  | \                    /
%       \        /
      
dpa = CT_A^-1 * (qvA - Aa*dxA - qvlk);

%       /        \
%       |   1    | /                    \
% dpB = | ------ | | Ab*dx + qvex - qvB | 
%       |  CT_B  | \                    /
%       \        /
      
dpb = CT_B^-1 * (Ab*dxA + qvlk - qvB);
end

dpA = dpa;
dpB = dpb;

== matlab function hydraulic_act_systems/HydroActuator + lever arm KNEE/Joint q2 --> x_Knee ==
  data: a2 parameter; x_Knee output; b2 parameter; e21 parameter; e22 parameter; Lcyl parameter; q2 input
function x_Knee = fcn(a2,b2,e21,e22,Lcyl,q2)
%#codegen
%Knee
ang2 = pi + q2 - e21 - e22;
c2 = sqrt(a2^2 + b2^2 - 2*a2*b2*cos(ang2));
x_Knee = c2-Lcyl;

== matlab function hydraulic_act_systems/HydroActuator + lever arm KNEE/Hydraulic system/Cylinder HOERBIGER LB6 1610 0080 4M/Mechanical equation ==
  data: Delta_F output; dxA input; pA input; pB input; fv input; Aa parameter; Ab parameter
function Delta_F = fcn(dxA, pA, pB, fv, Aa, Ab)
%#codegen

FH  = pA*Aa - pB*Ab;     % N - Hydraulic force
Ffr = fv*dxA;            % N - Friction force (Viscous)
Delta_F  = FH - Ffr;     % m/s2 - Acceleration

== matlab function hydraulic_act_systems/HydroActuator + lever arm KNEE/Hydraulic system/Servovalve MOOG E024-177LA/Flow rate equation + dead zone ==
  data I settings: updateMethod=SF_CONTINUOUS_TIME_DATA
  data qvA settings: updateMethod=SF_CONTINUOUS_TIME_DATA
  data qvB settings: updateMethod=SF_CONTINUOUS_TIME_DATA
  data: I input; qvA output; qvB output; In parameter; Kva parameter; Kvb parameter; KvlkA parameter; KvlkB parameter; up_dz parameter; lw_dz parameter; ps parameter; pt parameter; pA input; pB input
function [qvA , qvB] = fcn(I, In, Kva, Kvb, KvlkA, KvlkB,up_dz, lw_dz, ps, pt, pA, pB)

if (I>=up_dz) && (I<=In),
    qvA = (Kva*(I/In) + KvlkA) * sign(ps-pA)*sqrt(abs(ps-pA)) - KvlkA*sign(pA-pt)*sqrt(abs(pA-pt)) ;
    qvB = (Kvb*(I/In) + KvlkB) * sign(pB-pt)*sqrt(abs(pB-pt)) - KvlkB*sign(ps-pB)*sqrt(abs(ps-pB)) ;
elseif (I>=-In) && (I<=lw_dz), 
    qvA = KvlkA*sign(ps-pA)*sqrt(abs(ps-pA)) - (Kva*(abs(I)/In) + KvlkA) * sign(pA-pt)*sqrt(abs(pA-pt));
     qvB = KvlkB*sign(pB-pt)*sqrt(abs(pB-pt)) - (Kvb*(abs(I)/In) + KvlkB) * sign(ps-pB)*sqrt(abs(ps-pB));
else
    qvA = 0;
    qvB = 0;
end
end

== matlab function hydraulic_act_systems/HydroActuator + lever arm HIP/Joint q1 --> x_Hip   ==
  data: a1 parameter; x_Hip output; b1 parameter; e11 parameter; e12 parameter; Lcyl parameter; q1 input
function x_Hip = fcn(a1,b1,e11,e12,Lcyl,q1)
%#codegen

%Hip
ang1 = pi/2 - q1 + e11 - e12; 
c1 = sqrt(a1^2 + b1^2 - 2*a1*b1*cos(ang1));

x_Hip = c1-Lcyl;

== matlab function hydraulic_act_systems/HydActuator + lever arm HIP 2nd Approach/Joint q1 --> x_Hip   ==
  data: a1 parameter; x_Hip output; b1 parameter; e11 parameter; e12 parameter; Lcyl parameter; q1 input
function x_Hip = fcn(a1,b1,e11,e12,Lcyl,q1)
%#codegen

%Hip
ang1 = pi/2 - q1 + e11 - e12; 
c1 = sqrt(a1^2 + b1^2 - 2*a1*b1*cos(ang1));

x_Hip = c1-Lcyl;

== matlab function hydraulic_act_systems/HydActuator + lever arm HIP 2nd Approach/lever arm Hip ==
  data: a1 parameter; T_Hip output; b1 parameter; e11 parameter; e12 parameter; F1 input; q1 input
function T_Hip = fcn(a1,b1,e11,e12,F1,q1)
%#codegen

%Hip
ang1 = pi/2 - q1 + e11 - e12; 
c1 = sqrt(a1^2 + b1^2 - 2*a1*b1*cos(ang1));
L1 = a1*sin(acos((a1^2+c1^2-b1^2)/(2*a1*c1)));
T_Hip = F1*L1;

== matlab function hydraulic_act_systems/HydroActuator + lever arm KNEE 2nd Approach/Joint q2 --> x_Knee ==
  data: a2 parameter; x_Knee output; b2 parameter; e21 parameter; e22 parameter; Lcyl parameter; q2 input
function x_Knee = fcn(a2,b2,e21,e22,Lcyl,q2)
%#codegen
%Knee
ang2 = pi + q2 - e21 - e22;
c2 = sqrt(a2^2 + b2^2 - 2*a2*b2*cos(ang2));
x_Knee = c2-Lcyl;

== matlab function hydraulic_act_systems/HydroActuator + lever arm HIP/lever arm Hip ==
  data: a1 parameter; T_Hip output; b1 parameter; e11 parameter; e12 parameter; F1 input; q1 input
function T_Hip = fcn(a1,b1,e11,e12,F1,q1)
%#codegen

%Hip
ang1 = pi/2 - q1 + e11 - e12; 
c1 = sqrt(a1^2 + b1^2 - 2*a1*b1*cos(ang1));
L1 = a1*sin(acos((a1^2+c1^2-b1^2)/(2*a1*c1)));
T_Hip = F1*L1;

== matlab function hydraulic_act_systems/HydroActuator + lever arm KNEE/lever arm Knee ==
  data: a2 parameter; T_Knee output; b2 parameter; e21 parameter; e22 parameter; q2 input; F2 input
function T_Knee = fcn(a2,b2,e21,e22,q2,F2)
%#codegen

%Knee
ang2 = pi + q2 - e21 - e22;
c2 = sqrt(a2^2 + b2^2 - 2*a2*b2*cos(ang2));
L2 = a2*sin(acos((a2^2+c2^2-b2^2)/(2*a2*c2)));
T_Knee = F2*L2;

== matlab function hydraulic_act_systems/HydroActuator + lever arm KNEE 2nd Approach/lever arm Knee ==
  data: a2 parameter; T_Knee output; b2 parameter; e21 parameter; e22 parameter; q2 input; F2 input
function T_Knee = fcn(a2,b2,e21,e22,q2,F2)
%#codegen

%Knee
ang2 = pi + q2 - e21 - e22;
c2 = sqrt(a2^2 + b2^2 - 2*a2*b2*cos(ang2));
L2 = a2*sin(acos((a2^2+c2^2-b2^2)/(2*a2*c2)));
T_Knee = F2*L2;

== matlab function hydraulic_act_systems/HydroActuator + lever arm KNEE 2nd Approach/Hydraulic system/Cylinder HOERBIGER LB6 1610 0080 4M/Continuity equation ==
  data: xA input; dpA output; dpB output; dxA input; qvA input; qvB input; pA input; pB input; leak parameter; V0A parameter; V0B parameter; Aa parameter; Ab parameter; L parameter; beta parameter; n parameter; V0 parameter; P0 parameter; acc parameter
function [dpA,dpB] = fcn(xA, dxA, qvA, qvB, pA, pB, leak, V0A, V0B, Aa, Ab, L, beta, n, V0, P0, acc)

pC = pA - pB;   % Pressao de carga [Pa]

qvlk = leak * pC;
dpa = 0;
dpb = 0;

if acc == 0,
%       /              \
%       |     beta     | /                    \
% dpA = | ------------ | | qvA - Aa*dx - qvex | 
%       |  Va0 + Aa*x  | \                    /
%       \              /
      
dpa = (beta/(V0A + Aa*xA)) * (qvA - Aa*dxA - qvlk);

%       /                  \
%       |     beta         | /                    \
% dpB = | ---------------- | | Ab*dx + qvex - qvB | 
%       | Vb0 + Ab*(L - x) | \                    /
%       \                  /
      
dpb = (beta/(V0B + Ab*(L-xA))) * (Ab*dxA + qvlk - qvB);

elseif acc == 1,
    
CA_A  = (V0A + Aa*xA) / beta;                      % Capacitancia hidráulica do atuador [m^3/Pa]
CAC_A = (V0*P0^(1/n))/(n* (pA+1e5)^((n+1)/n));     % Capacitancia hidráulica do acumulador [m^3/Pa]
CA_B  = (V0B + Ab*(L-xA)) / beta;                  % Capacitancia hidráulica do atuador [m^3/Pa]
CAC_B = (V0*P0^(1/n))/(n* (pB+1e5)^((n+1)/n));     % Capacitancia hidráulica do acumulador [m^3/Pa]

CT_A  = CA_A + CAC_A;                              % Capacitancia total em A
CT_B  = CA_B + CAC_B;                              % Capacitancia total em B 


%       /        \
%       |   1    | /                    \
% dpA = | ------ | | qvA - Aa*dx - qvex | 
%       |  CT_A  | \                    /
%       \        /
      
dpa = CT_A^-1 * (qvA - Aa*dxA - qvlk);

%       /        \
%       |   1    | /                    \
% dpB = | ------ | | Ab*dx + qvex - qvB | 
%       |  CT_B  | \                    /
%       \        /
      
dpb = CT_B^-1 * (Ab*dxA + qvlk - qvB);
end

dpA = dpa;
dpB = dpb;

== matlab function hydraulic_act_systems/HydroActuator + lever arm KNEE 2nd Approach/Hydraulic system/Cylinder HOERBIGER LB6 1610 0080 4M/Mechanical equation ==
  data: Fe output; xL input; xA input; dxA input; ddx output; pA input; pB input; fv input; Aa parameter; Ab parameter; Ks parameter; Mp parameter; noise parameter
function [Fe, ddx] = fcn(xL, xA, dxA, pA, pB, fv, Aa, Ab, Ks, Mp, noise)
%#codegen

FH  = pA*Aa - pB*Ab;                % N - Hydraulic force
Ffr = fv*dxA;                       % N - Friction force (Viscous)
Fe  = Ks*(xA - xL) + noise*randn(1);% N - Force measured by the sensor + noise
ddx = (FH - Ffr - Fe)/Mp;        % m/s2 - Acceleration

== matlab function hydraulic_act_systems/HydroActuator + lever arm KNEE 2nd Approach/Hydraulic system/Servovalve MOOG E024-177LA/Flow rate equation + dead zone ==
  data I settings: updateMethod=SF_CONTINUOUS_TIME_DATA
  data qvA settings: updateMethod=SF_CONTINUOUS_TIME_DATA
  data qvB settings: updateMethod=SF_CONTINUOUS_TIME_DATA
  data: I input; qvA output; qvB output; In parameter; Kva parameter; Kvb parameter; KvlkA parameter; KvlkB parameter; up_dz parameter; lw_dz parameter; ps parameter; pt parameter; pA input; pB input
function [qvA , qvB] = fcn(I, In, Kva, Kvb, KvlkA, KvlkB,up_dz, lw_dz, ps, pt, pA, pB)

if (I>=up_dz) && (I<=In),
    qvA = (Kva*(I/In) + KvlkA) * sign(ps-pA)*sqrt(abs(ps-pA)) - KvlkA*sign(pA-pt)*sqrt(abs(pA-pt)) ;
    qvB = (Kvb*(I/In) + KvlkB) * sign(pB-pt)*sqrt(abs(pB-pt)) - KvlkB*sign(ps-pB)*sqrt(abs(ps-pB)) ;
elseif (I>=-In) && (I<=lw_dz), 
    qvA = KvlkA*sign(ps-pA)*sqrt(abs(ps-pA)) - (Kva*(abs(I)/In) + KvlkA) * sign(pA-pt)*sqrt(abs(pA-pt));
     qvB = KvlkB*sign(pB-pt)*sqrt(abs(pB-pt)) - (Kvb*(abs(I)/In) + KvlkB) * sign(ps-pB)*sqrt(abs(ps-pB));
else
    qvA = 0;
    qvB = 0;
end
end
